simulink model "Rover"  (R2023b)
settings: Solver=FixedStepDiscrete  StartTime=0.0  StopTime=1000  RelTol=1e-3  EnableMultiTasking=on
model workspace (MAT data in the model file):
  state_1 = 0
(part 2 of 2)

== stateflow chart Rover/Chart ==
  settings: updateMethod=DISCRETE  sampleTime=0.001
  state BOARD_1 [parallel]
    settings: executionOrder=1
    state WAITING_INITIALIZATION
      en:
      init_encoder();
      init_encoder();
      init_encoder();
      init_encoder();
      init_motor_driver();
      init_motor_driver();
    state INITIALIZED
    state WORKING
      state LED_CONTROLLER [parallel]
        settings: executionOrder=3
        state SINGLE
          state RIGHT [parallel]
            settings: executionOrder=1
            state OFF
            state ON
            (default) -> BOARD_1.WORKING.LED_CONTROLLER.SINGLE.RIGHT.OFF
            BOARD_1.WORKING.LED_CONTROLLER.SINGLE.RIGHT.ON -> BOARD_1.WORKING.LED_CONTROLLER.SINGLE.RIGHT.OFF : [RH_LED_OFF]
                | {rh_led.off()}
            BOARD_1.WORKING.LED_CONTROLLER.SINGLE.RIGHT.OFF -> BOARD_1.WORKING.LED_CONTROLLER.SINGLE.RIGHT.ON : [RH_LED_ON]
                | {rh_led.on()}
          state LEFT [parallel]
            settings: executionOrder=2
            state OFF
            state ON
            (default) -> BOARD_1.WORKING.LED_CONTROLLER.SINGLE.LEFT.OFF
            BOARD_1.WORKING.LED_CONTROLLER.SINGLE.LEFT.ON -> BOARD_1.WORKING.LED_CONTROLLER.SINGLE.LEFT.OFF : [LH_LED_OFF]
                | {lh_led.off()}
            BOARD_1.WORKING.LED_CONTROLLER.SINGLE.LEFT.OFF -> BOARD_1.WORKING.LED_CONTROLLER.SINGLE.LEFT.ON : [LH_LED_ON]
                | {lh_led.on()}
        state rh_led [group]
        state BOTH
          state WAITING_ON
          state ON
            en:
            rh_led.on();
            lh_led.on()
          state WAITING_OFF
          (default) -> WAITING_ON
          WAITING_ON -> BOARD_1.WORKING.LED_CONTROLLER.BOTH.ON : [LEDS_BTN_RELEASED]
          BOARD_1.WORKING.LED_CONTROLLER.BOTH.ON -> WAITING_OFF : [LEDS_BTN_PRESSED]
        state lh_led [group]
        (default) -> SINGLE
        SINGLE -> BOTH : [LEDS_BTN_PRESSED]
        WAITING_OFF -> SINGLE : [LEDS_BTN_RELEASED]
            | {rh_led.off(); lh_led.off()}
      state STATE_UPDATING [parallel]
        settings: executionOrder=1
        state UPDATE
          en:
          rpm_motors = read_rpm();
          motors_direction = read_motors_direction();
          temperature_B1 = read_temperature();
        (default) -> BOARD_1.WORKING.STATE_UPDATING.UPDATE
        BOARD_1.WORKING.STATE_UPDATING.UPDATE -> BOARD_1.WORKING.STATE_UPDATING.UPDATE : after(READ_PERIOD,  msec)
      state COMM_PROCESS_DECISION [parallel]
        settings: executionOrder=2
        state WAITING_FOR_RTR [parallel]
          settings: executionOrder=2
          state WAITING_BOARD_2
          state BOARD_2_READY
          (default) -> WAITING_BOARD_2
          WAITING_BOARD_2 -> BOARD_2_READY : [B2_RTR]
          BOARD_2_READY -> WAITING_BOARD_2 : [RESET]
        state COMMUNICATION [parallel]
          settings: executionOrder=1
          state TRANSMITTING_TO_B2_1
            en:
            B1_state = capture_state(rpm_motors, motors_direction, ...
            temperature_B1);
          state WAITING_B2_RTR_1
            en: has_retransmitted = false;
          state WAITING_B2_TRANSMISSION_1
            en: send(B1_RTR, BOARD_2)
          state PROCESSING
            en:
            encoder_status = check_encoder(rpm_motors);
            motor_driver_status = check_temperature(check_temperature_values(temperature_B1, temperature_B2));
            mpu_status = check_mpu(control_value, MPU_MASK);
            joypad_status = check_joypad(control_value, JOYPAD_MASK);
            sabertooth_status = check_motor_driver(motors_direction, current_state);
          state res = check_temperature(temperature_status) [function]
            (default) -> (junction 3062)
            (junction 3062) -> (junction 3053) [order 1] : [temperature_status == TEMPERATURE_STATUS.CRITICAL]
                | {res = TEMPERATURE_STATUS.CRITICAL;
                | temperature_out = 2;}
            (junction 3062) -> (junction 3063) [order 2] : [temperature_status == TEMPERATURE_STATUS.NORMAL && ...
                | (in(TEMPERATURE_CONTROLLER.TIMER_STARTED) || ...
                | in(TEMPERATURE_CONTROLLER.TIMER_ELAPSED))]
                | {send(RESET_TEMP_TIMER, TEMPERATURE_CONTROLLER);
                | res = TEMPERATURE_STATUS.NORMAL;
                | temperature_out = 0;}
            (junction 3062) -> (junction 3051) [order 3]
            (junction 3051) -> (junction 3067) [order 1] : [in(TEMPERATURE_CONTROLLER.TIMER_ELAPSED)]
                | {res =TEMPERATURE_STATUS.ABOVE_NORMAL;
                | temperature_out = 1;}
            (junction 3051) -> (junction 3055) [order 2] : [temperature_status == TEMPERATURE_STATUS.ABOVE_NORMAL && ...
                | in(TEMPERATURE_CONTROLLER.TIMER_STOP)]
                | {send(START_TEMP_TIMER, TEMPERATURE_CONTROLLER);
                | res = TEMPERATURE_STATUS.NORMAL;
                | temperature_out = 0;}
            (junction 3051) -> (junction 3056) [order 3] : {res = TEMPERATURE_STATUS.NORMAL;
                | temperature_out = 0;}
          state WAITING_B2_RTR_2
          state TRANSMITTING_TO_B2_2
            en: B1_intention = [double(next_state), ...
            double(degraded), double(braking)];
          state WAITING_B2_TRANSMISSION_2
            en: send(B1_RTR, BOARD_2)
          (junction 1462) -> TRANSMITTING_TO_B2_1 [order 2] : [~has_retransmitted]/{has_retransmitted = true;}
          (default) -> WAITING_B2_RTR_1
          WAITING_B2_RTR_1 -> TRANSMITTING_TO_B2_1 [order 1] : [in(WAITING_FOR_RTR.BOARD_2_READY)]
              | {send(RESET, WAITING_FOR_RTR)}
          TRANSMITTING_TO_B2_1 -> (junction 1462) [order 2] : after(COMM_TIMEOUT,msec)
          (junction 1462) -> (junction 3045) [order 1] : [has_retransmitted]
          (junction 1483) -> (junction 1462) [order 2]
          (junction 3045) -> (junction 1482)
          WAITING_B2_RTR_1 -> (junction 1484) [order 2] : after(B2_ALIVE, msec)
          (junction 3049) -> WAITING_B2_RTR_1
          TRANSMITTING_TO_B2_1 -> WAITING_B2_TRANSMISSION_1 [order 1] : [B2_ACK]{has_retransmitted = false;}
          WAITING_B2_TRANSMISSION_1 -> (junction 1482) [order 1] : after(COMM_TIMEOUT, msec)
          (junction 1482) -> (junction 3047)
          WAITING_B2_TRANSMISSION_1 -> BOARD_1.WORKING.COMM_PROCESS_DECISION.COMMUNICATION.PROCESSING [order 2] : [change(B2_state)]
              | {[obstacle_distances, accX, gyroZ, y_analog, x_analog, control_buttons, ...
              |     control_value, temperature_B2] = update_global_state(B2_state);
              | send(B1_ACK, BOARD_2)}
          BOARD_1.WORKING.COMM_PROCESS_DECISION.COMMUNICATION.PROCESSING -> (junction 1879)
          (junction 1879) -> (junction 1878) [order 1] : [encoder_status == ENCODER_STATUS.ENCODER_ERR || ...
              | joypad_status == JOYPAD_ERR || ...
              | sabertooth_status == SABERTOOTH_STATUS.SABERTOOTH_ERR || ...
              | motor_driver_status == TEMPERATURE_STATUS.CRITICAL]
              | {next_state = EMERGENCY;}
          (junction 1879) -> (junction 1886) [order 2]
          (junction 1878) -> (junction 1877)
          (junction 1886) -> (junction 1885) [order 1] : [(encoder_status ~= ENCODER_STATUS.ENCODER_ERR  && ...
              | encoder_status ~= ENCODER_STATUS.ENCODER_OK) || ...
              | mpu_status == MPU_STATUS.MPU_ERR || ...
              | motor_driver_status == TEMPERATURE_STATUS.ABOVE_NORMAL]
              | {degraded = DEGRADED_STATUS.ACTIVE;}
          (junction 1886) -> (junction 1882) [order 2]
          (junction 1885) -> (junction 1884)
          (junction 1882) -> (junction 1884) : {degraded = DEGRADED_STATUS.INACTIVE;}
          (junction 1884) -> (junction 1877) : {next_state = update_next_state(current_state, y_analog, ...
              |         x_analog, obstacle_distances, control_buttons);}
          (junction 1877) -> WAITING_B2_RTR_2
          WAITING_B2_RTR_2 -> (junction 3047) [order 1] : after(COMM_TIMEOUT, msec)
          (junction 3047) -> (junction 3041)
          WAITING_B2_RTR_2 -> TRANSMITTING_TO_B2_2 [order 2] : [in(WAITING_FOR_RTR.BOARD_2_READY)]
              | {send(RESET, WAITING_FOR_RTR)}
          (junction 1483) -> TRANSMITTING_TO_B2_2 [order 1] : [~has_retransmitted]/{has_retransmitted = true;}
          TRANSMITTING_TO_B2_2 -> (junction 1483) [order 2] : after(COMM_TIMEOUT, msec)
          TRANSMITTING_TO_B2_2 -> WAITING_B2_TRANSMISSION_2 [order 1] : [B2_ACK]
          WAITING_B2_TRANSMISSION_2 -> (junction 3041) [order 2] : after(COMM_TIMEOUT, msec)
          (junction 3041) -> (junction 3042)
          WAITING_B2_TRANSMISSION_2 -> (junction 1475) [order 1] : change(B2_intention)
              | {send(B1_ACK, BOARD_2)}
          (junction 1475) -> (junction 3049) [order 1] : [all(B1_intention == B2_intention)]
              | {current_state = ROVER_STATE(B1_intention(1));
              | led.action()}
          (junction 1475) -> (junction 3042) [order 2]
          (junction 3042) -> (junction 1471)
          (junction 1484) -> (junction 1471)
        state TEMPERATURE_CONTROLLER [parallel]
          settings: executionOrder=3
          state TIMER_STOP
          state TIMER_STARTED
          state TIMER_ELAPSED
          (default) -> BOARD_1.WORKING.COMM_PROCESS_DECISION.TEMPERATURE_CONTROLLER.TIMER_STOP
          BOARD_1.WORKING.COMM_PROCESS_DECISION.TEMPERATURE_CONTROLLER.TIMER_STOP -> BOARD_1.WORKING.COMM_PROCESS_DECISION.TEMPERATURE_CONTROLLER.TIMER_STARTED : [START_TEMP_TIMER]
          BOARD_1.WORKING.COMM_PROCESS_DECISION.TEMPERATURE_CONTROLLER.TIMER_STARTED -> BOARD_1.WORKING.COMM_PROCESS_DECISION.TEMPERATURE_CONTROLLER.TIMER_STOP [order 2] : [RESET_TEMP_TIMER]
          BOARD_1.WORKING.COMM_PROCESS_DECISION.TEMPERATURE_CONTROLLER.TIMER_ELAPSED -> BOARD_1.WORKING.COMM_PROCESS_DECISION.TEMPERATURE_CONTROLLER.TIMER_STOP : [RESET_TEMP_TIMER]
          BOARD_1.WORKING.COMM_PROCESS_DECISION.TEMPERATURE_CONTROLLER.TIMER_STARTED -> BOARD_1.WORKING.COMM_PROCESS_DECISION.TEMPERATURE_CONTROLLER.TIMER_ELAPSED [order 1] : [after(TEMP_TIMEOUT, sec)]
        state led [group]
          state rh_led_action [function]
            (default) -> (junction 2941)
            (junction 2941) -> (junction 2942) [order 1] : [bitand(control_buttons, RH_LED_MASK) == 0]
            (junction 2941) -> (junction 2943) [order 2] : {send(RH_LED_ON, ...
                | LED_CONTROLLER)}
            (junction 2942) -> (junction 2944) : {send(RH_LED_OFF, ...
                | LED_CONTROLLER);}
            (junction 2944) -> (junction 2943)
            (junction 2943) -> (junction 2945)
          state lh_led_action [function]
            (default) -> (junction 2955)
            (junction 2955) -> (junction 2946) [order 1] : [bitand(control_buttons, LH_LED_MASK) == 0]
            (junction 2955) -> (junction 2948) [order 2] : {send(LH_LED_ON, ...
                | LED_CONTROLLER)}
            (junction 2946) -> (junction 2949) : {send(LH_LED_OFF, ...
                | LED_CONTROLLER);}
            (junction 2949) -> (junction 2948)
            (junction 2948) -> (junction 2956)
          state action [function]
            (default) -> (junction 2958)
            (junction 2958) -> (junction 2960) [order 1] : [bitand(control_buttons, BOTH_LED_MASK) ~= 0]
            (junction 2958) -> (junction 2964) [order 2] : {send(LEDS_BTN_RELEASED, ...
                | LED_CONTROLLER)}
            (junction 2960) -> (junction 2962) : {send(LEDS_BTN_PRESSED, ...
                | LED_CONTROLLER)}
            (junction 2962) -> (junction 2964)
            (junction 2964) -> (junction 2967) : {rh_led_action();
                | lh_led_action()}
    state EMERGENCY
      en:
      rover_status_out = 2;
      % fermare i motori
    (default) -> BOARD_1.WAITING_INITIALIZATION
    BOARD_1.WAITING_INITIALIZATION -> BOARD_1.INITIALIZED : after(1, msec)
    BOARD_1.INITIALIZED -> BOARD_1.WORKING : [in(BOARD_2.INITIALIZED) || in(BOARD_2.WORKING)]
    (junction 1471) -> BOARD_1.EMERGENCY
  state BOARD_2 [parallel]
    settings: executionOrder=2
    state WAITING_INITIALIZATION
      en:
      init_motor_driver();
      init_motor_driver();
      init_ps2x();
      init_ultrasonic_sensors();
      init_mpu();
    state INITIALIZED
    state WORKING
      state STATE_UPDATING [parallel]
        settings: executionOrder=1
        state UPDATE
          en:
          obstacle_distances = read_ultrasonic_sensors();
          [accX, gyroZ] = read_mpu();
          [y_analog, x_analog, control_buttons, control_value] = read_joypad(control_buttons);
          temperature_B2 = read_temperature();
        (default) -> BOARD_2.WORKING.STATE_UPDATING.UPDATE
        BOARD_2.WORKING.STATE_UPDATING.UPDATE -> BOARD_2.WORKING.STATE_UPDATING.UPDATE : after(READ_PERIOD, msec)
      state EXECUTION [parallel]
        settings: executionOrder=3
        state DRIVE
          state MODE [parallel]
            settings: executionOrder=1
            state NORMAL
              en:
              rover_status_out = 0;
              % settare velocità
              % massima
            state DEGRADED
              en:
              rover_status_out = 1;
              % settare velocità
              % massima
            (default) -> NORMAL
            DEGRADED -> NORMAL : [MINOR_ERROR_RES]
            NORMAL -> DEGRADED : [MINOR_ERROR]
          state EXECUTE [parallel]
            settings: executionOrder=2
            state MOVE
              state STOP
                state SMOOTH_STOP
                  en:
                  stop.smooth()
                state HARD_STOP
                  state BRAKE
                    en:
                    stop.hard()
                  state ROTATION
                    state ROTATE_RIGHT
                      en:
                      go.right()
                    state ROTATE_LEFT
                      en:
                      go.left()
                    (default) -> (junction 2721)
                    (junction 2721) -> ROTATE_RIGHT [order 1] : [obstacle ~= OBSTACLE_DIR.RIGHT_SIDE]
                    (junction 2721) -> ROTATE_LEFT [order 2]
                  (junction 2736) -> BRAKE [order 2]
                  (default) -> (junction 2736)
                  (junction 2736) -> BOARD_2.WORKING.EXECUTION.DRIVE.EXECUTE.MOVE.STOP.HARD_STOP.ROTATION [order 1] : [obstacle ~= OBSTACLE_DIR.LEFT_RIGHT && ...
                      | obstacle ~= OBSTACLE_DIR.NOTONE]
                  BOARD_2.WORKING.EXECUTION.DRIVE.EXECUTE.MOVE.STOP.HARD_STOP.ROTATION -> BRAKE : [gyroZ >= 90]
                (default) -> (junction 2730)
                (junction 2730) -> SMOOTH_STOP [order 1] : [braking == SMOOTH]
                (junction 2730) -> HARD_STOP [order 2]
              state BACKWARD
                en:
                go.backward()
              state FORWARD
                en:
                go.ahead()
              state FORWARD_RIGHT
                en:
                go.forward_right()
              state FORWARD_LEFT
                en:
                go.forward_left()
              state RIGHT
                en:
                go.right()
              state LEFT
                en:
                go.left()
              state ALT_BACKWARD
                state ROTATION
                  en:
                  go.right();
                state ROTATED
                  en:
                  stop.hard();
                  control_buttons = 0
                BOARD_2.WORKING.EXECUTION.DRIVE.EXECUTE.MOVE.ALT_BACKWARD.ROTATION -> ROTATED : [gyroZ >= 180]
                (default) -> BOARD_2.WORKING.EXECUTION.DRIVE.EXECUTE.MOVE.ALT_BACKWARD.ROTATION
            state IDLE
            (junction 1424) -> (junction 1425)
            (junction 1425) -> IDLE
            STOP -> (junction 1424) : [all(rpm_motors == 0)]
            (default) -> IDLE
            MOVE -> (junction 1420)
            (junction 1420) -> (junction 1415)
            IDLE -> (junction 1413)
            (junction 1415) -> STOP [order 1] : [IDLE]
            (junction 1415) -> (junction 1427) [order 2]
            (junction 1413) -> (junction 1427)
            (junction 1427) -> BACKWARD [order 1] : [BACKWARD]
            (junction 1427) -> (junction 1414) [order 2]
            (junction 1414) -> FORWARD [order 1] : [FORWARD]
            (junction 1414) -> (junction 1421) [order 2]
            (junction 1421) -> (junction 2085) [order 1] : [FORWARD_RIGHT]
            (junction 2085) -> FORWARD_RIGHT [order 2]
            (junction 1421) -> (junction 1432) [order 2]
            (junction 2085) -> (junction 2087) [order 1] : [in(MODE.DEGRADED)]
            (junction 1432) -> (junction 2090) [order 1] : [FORWARD_LEFT]
            (junction 2090) -> FORWARD_LEFT [order 2]
            (junction 1432) -> (junction 1428) [order 2]
            (junction 2090) -> (junction 2092) [order 1] : [in(MODE.DEGRADED)]
            (junction 1428) -> (junction 2087) [order 1] : [RIGHT]
            (junction 2087) -> BOARD_2.WORKING.EXECUTION.DRIVE.EXECUTE.MOVE.RIGHT
            (junction 1428) -> (junction 1408) [order 2]
            (junction 1408) -> (junction 2092) [order 1] : [LEFT]
            (junction 2092) -> BOARD_2.WORKING.EXECUTION.DRIVE.EXECUTE.MOVE.LEFT
            (junction 1408) -> (junction 2675) [order 2]
            (junction 2675) -> ALT_BACKWARD : [ALT_BACKWARD]
          state go [group]
          state stop [group]
      state COMM_PROCESS_DECISION [parallel]
        settings: executionOrder=2
        state COMMUNICATION [parallel]
          settings: executionOrder=1
          state WAITING_FOR_COMMUNICATION
            en: has_retransmitted = false;
          state WAITING_B1_TRANSMISSION_1
            en: send(B2_RTR, BOARD_1)
          state WAITING_B1_RTR_1
            en:
            [rpm_motors, motors_direction, temperature_B1] = update_global_state(B1_state);
          state res = check_temperature(temperature_status) [function]
            (default) -> (junction 2144)
            (junction 2144) -> (junction 2143) [order 1] : [temperature_status == TEMPERATURE_STATUS.CRITICAL]
                | {res = TEMPERATURE_STATUS.CRITICAL;
                | temperature_out = 2;}
            (junction 2144) -> (junction 2546) [order 2] : [temperature_status == TEMPERATURE_STATUS.NORMAL && ...
                | (in(TEMPERATURE_CONTROLLER.TIMER_STARTED) || ...
                | in(TEMPERATURE_CONTROLLER.TIMER_ELAPSED))]
                | {send(RESET_TEMP_TIMER, TEMPERATURE_CONTROLLER);
                | res = TEMPERATURE_STATUS.NORMAL;
                | temperature_out = 0;}
            (junction 2144) -> (junction 2138) [order 3]
            (junction 2138) -> (junction 2134) [order 1] : [in(TEMPERATURE_CONTROLLER.TIMER_ELAPSED)]
                | {res =TEMPERATURE_STATUS.ABOVE_NORMAL;
                | temperature_out = 1;}
            (junction 2138) -> (junction 2145) [order 2] : [temperature_status == TEMPERATURE_STATUS.ABOVE_NORMAL && ...
                | in(TEMPERATURE_CONTROLLER.TIMER_STOP)]
                | {send(START_TEMP_TIMER, TEMPERATURE_CONTROLLER);
                | res = TEMPERATURE_STATUS.NORMAL;
                | temperature_out = 0;}
            (junction 2138) -> (junction 2139) [order 3] : {res = TEMPERATURE_STATUS.NORMAL;
                | temperature_out = 0;}
          state TRANSMITTING_TO_B1_1
            en:
            B2_state  = capture_state(obstacle_distances, accX, gyroZ, y_analog, ...
            x_analog, control_buttons, control_value, temperature_B2);
          state PROCESSING
            en:
            encoder_status = check_encoder(rpm_motors);
            temperature_status = check_temperature(check_temperature_values(temperature_B1, temperature_B2));
            mpu_status = check_mpu(control_value, MPU_MASK);
            joypad_status = check_joypad(control_value, JOYPAD_MASK);
            motor_driver_status = check_motor_driver(motors_direction, current_state);
          state WAITING_B1_TRANSMISSION_2
            en: send(B2_RTR, BOARD_1)
          state WAITING_B1_RTR_2
            en:
            if degraded == DEGRADED_STATUS.ACTIVE
            send(MINOR_ERROR, EXECUTION)
            else
            send(MINOR_ERROR_RES, EXECUTION)
            end
            current_state = next_state;
            action
          state COMMUNICATION_TIMEOUT
          state TRANSMITTING_TO_B1_2
            en: B2_intention = [double(next_state), ...
            double(degraded), double(braking)];
          (default) -> WAITING_FOR_COMMUNICATION
          WAITING_B1_TRANSMISSION_1 -> (junction 1528) [order 2] : after(COMM_TIMEOUT, msec)
          WAITING_FOR_COMMUNICATION -> WAITING_B1_TRANSMISSION_1 : [after(COMM_PERIOD, msec)]
          (junction 1528) -> (junction 3070)
          WAITING_B1_TRANSMISSION_1 -> WAITING_B1_RTR_1 [order 1] : [change(B1_state)]
              | {send(B2_ACK, BOARD_1)}
          (junction 3078) -> WAITING_FOR_COMMUNICATION
          WAITING_B1_RTR_1 -> (junction 3070) [order 1] : after(COMM_TIMEOUT, msec)
          (junction 3070) -> (junction 1529)
          WAITING_B1_RTR_1 -> TRANSMITTING_TO_B1_1 [order 2] : [in(WAITING_FOR_RTR.BOARD_1_READY)]
              | {send(RESET, WAITING_FOR_RTR)}
          (junction 1509) -> TRANSMITTING_TO_B1_1 [order 1] : [~has_retransmitted]{has_retransmitted = true;}
          TRANSMITTING_TO_B1_1 -> (junction 1509) [order 2] : after(COMM_TIMEOUT, msec)
          (junction 1509) -> (junction 3074) [order 2] : [has_retransmitted]
          TRANSMITTING_TO_B1_1 -> BOARD_2.WORKING.COMM_PROCESS_DECISION.COMMUNICATION.PROCESSING [order 1] : [B1_ACK]{has_retransmitted = false;}
          BOARD_2.WORKING.COMM_PROCESS_DECISION.COMMUNICATION.PROCESSING -> (junction 1729)
          (junction 1729) -> (junction 1731) [order 1] : [encoder_status == ENCODER_STATUS.ENCODER_ERR || ...
              | joypad_status == JOYPAD_STATUS.JOYPAD_ERR || ...
              | motor_driver_status == SABERTOOTH_STATUS.SABERTOOTH_ERR || ...
              | temperature_status == TEMPERATURE_STATUS.CRITICAL]
              | {next_state = EMERGENCY;}
          (junction 1729) -> (junction 1733) [order 2]
          (junction 1731) -> (junction 1744)
          (junction 1733) -> (junction 1735) [order 1] : [(encoder_status ~= ENCODER_STATUS.ENCODER_ERR  && ...
              | encoder_status ~= ENCODER_STATUS.ENCODER_OK) || ...
              | mpu_status == MPU_STATUS.MPU_ERR || ...
              | temperature_status == TEMPERATURE_STATUS.ABOVE_NORMAL]
              | {degraded = DEGRADED_STATUS.ACTIVE;}
          (junction 1733) -> (junction 1738) [order 2]
          (junction 1735) -> (junction 1740)
          (junction 1738) -> (junction 1740) : {degraded = DEGRADED_STATUS.INACTIVE;}
          (junction 1740) -> (junction 1744) : {next_state = update_next_state(current_state, y_analog, ...
              |         x_analog, obstacle_distances, control_buttons);
              | obstacle = nearby_obstacle_direction(obstacle_distances);}
          (junction 1744) -> WAITING_B1_TRANSMISSION_2
          WAITING_B1_TRANSMISSION_2 -> (junction 3074) [order 1] : after(COMM_TIMEOUT, msec)
          (junction 3074) -> (junction 1501)
          WAITING_B1_TRANSMISSION_2 -> (junction 2076) [order 2] : [change(B1_intention)]
              | {send(B2_ACK, BOARD_1)}
          (junction 2076) -> (junction 3068) [order 1] : [all(B1_intention ~= [double(next_state), double(degraded), ...
              | double(braking)]) || next_state == EMERGENCY]
          (junction 2076) -> WAITING_B1_RTR_2 [order 2]
          WAITING_B1_RTR_2 -> (junction 1501) [order 1] : [after(COMM_TIMEOUT, msec)]
          (junction 1529) -> (junction 1501)
          (junction 3076) -> (junction 1501)
          (junction 1501) -> COMMUNICATION_TIMEOUT : {send(ACTIVE, SINGLE_BOARD);
              | send(MINOR_ERROR, EXECUTION)}
          (junction 1505) -> (junction 3076) [order 2]
          WAITING_B1_RTR_2 -> TRANSMITTING_TO_B1_2 [order 2] : [in(WAITING_FOR_RTR.BOARD_1_READY)]
              | {send(RESET, WAITING_FOR_RTR)}
          TRANSMITTING_TO_B1_2 -> (junction 1505) [order 2] : after(COMM_TIMEOUT, msec)
          (junction 1505) -> TRANSMITTING_TO_B1_2 [order 1] : [~has_retransmitted]{has_retransmitted = true;}
          TRANSMITTING_TO_B1_2 -> (junction 3078) [order 1] : [B1_ACK]
        state WAITING_FOR_RTR [parallel]
          settings: executionOrder=2
          state WAITING_BOARD_1
          state BOARD_1_READY
          (default) -> WAITING_BOARD_1
          WAITING_BOARD_1 -> BOARD_1_READY : [B1_RTR]
          BOARD_1_READY -> WAITING_BOARD_1 : [RESET]
        state TEMPERATURE_CONTROLLER [parallel]
          settings: executionOrder=3
          state TIMER_STOP
          state TIMER_STARTED
          state TIMER_ELAPSED
          (default) -> BOARD_2.WORKING.COMM_PROCESS_DECISION.TEMPERATURE_CONTROLLER.TIMER_STOP
          BOARD_2.WORKING.COMM_PROCESS_DECISION.TEMPERATURE_CONTROLLER.TIMER_STOP -> BOARD_2.WORKING.COMM_PROCESS_DECISION.TEMPERATURE_CONTROLLER.TIMER_STARTED : [START_TEMP_TIMER]
          BOARD_2.WORKING.COMM_PROCESS_DECISION.TEMPERATURE_CONTROLLER.TIMER_STARTED -> BOARD_2.WORKING.COMM_PROCESS_DECISION.TEMPERATURE_CONTROLLER.TIMER_STOP [order 2] : [RESET_TEMP_TIMER]
          BOARD_2.WORKING.COMM_PROCESS_DECISION.TEMPERATURE_CONTROLLER.TIMER_ELAPSED -> BOARD_2.WORKING.COMM_PROCESS_DECISION.TEMPERATURE_CONTROLLER.TIMER_STOP : [RESET_TEMP_TIMER]
          BOARD_2.WORKING.COMM_PROCESS_DECISION.TEMPERATURE_CONTROLLER.TIMER_STARTED -> BOARD_2.WORKING.COMM_PROCESS_DECISION.TEMPERATURE_CONTROLLER.TIMER_ELAPSED [order 1] : [after(TEMP_TIMEOUT, sec)]
      state action [function]
        (default) -> (junction 2798)
        (junction 2798) -> (junction 2799) [order 1] : [current_state == ROVER_STATE.IDLE]
        (junction 2798) -> (junction 2825) [order 2]
        (junction 2799) -> (junction 2833) : {send(IDLE, EXECUTION);}
        (junction 2833) -> (junction 2813)
        (junction 2813) -> (junction 2803)
        (junction 2825) -> (junction 2816) [order 1] : [current_state == ROVER_STATE.FORWARD]
        (junction 2825) -> (junction 2810) [order 2]
        (junction 2816) -> (junction 2802) : {send(FORWARD, EXECUTION);}
        (junction 2802) -> (junction 2803)
        (junction 2803) -> (junction 2807)
        (junction 2810) -> (junction 2827) [order 1] : [current_state == ROVER_STATE.LEFT]
        (junction 2810) -> (junction 2821) [order 2]
        (junction 2827) -> (junction 2801) : {send(LEFT, EXECUTION);}
        (junction 2801) -> (junction 2807)
        (junction 2807) -> (junction 2819)
        (junction 2821) -> (junction 2818) [order 1] : [current_state == ROVER_STATE.RIGHT]
        (junction 2821) -> (junction 2820) [order 2]
        (junction 2818) -> (junction 2806) : {send(RIGHT, EXECUTION);}
        (junction 2806) -> (junction 2819)
        (junction 2819) -> (junction 2828)
        (junction 2820) -> (junction 2804) [order 1] : [current_state == ROVER_STATE.FORWARD_RIGHT]
        (junction 2820) -> (junction 2826) [order 2]
        (junction 2804) -> (junction 2805) : {send(FORWARD_RIGHT, EXECUTION);}
        (junction 2805) -> (junction 2828)
        (junction 2828) -> (junction 2823)
        (junction 2826) -> (junction 2822) [order 1] : [current_state == ROVER_STATE.FORWARD_LEFT]
        (junction 2826) -> (junction 2811) [order 2]
        (junction 2822) -> (junction 2831) : {send(FORWARD_LEFT, EXECUTION);}
        (junction 2831) -> (junction 2823)
        (junction 2823) -> (junction 2808)
        (junction 2811) -> (junction 2824) [order 1] : [current_state == ROVER_STATE.BACKWARD]
        (junction 2811) -> (junction 2867) [order 2]
        (junction 2824) -> (junction 2817) : {send(BACKWARD, EXECUTION);}
        (junction 2817) -> (junction 2808)
        (junction 2808) -> (junction 2873)
        (junction 2867) -> (junction 2869) [order 1] : [current_state == ROVER_STATE.ALT_BACKWARD]
        (junction 2867) -> (junction 2829) [order 2] : {send(IDLE, EXECUTION);}
        (junction 2869) -> (junction 2871)
        (junction 2871) -> (junction 2873) : {send(ALT_BACKWARD, EXECUTION);}
        (junction 2873) -> (junction 2800)
        (junction 2800) -> (junction 2829)
        (junction 2829) -> (junction 2830)
      state SINGLE_BOARD [parallel]
        settings: executionOrder=4
        state PROCESSING
          en:
          if(temperature_B2 >= CRITICAL_TEMP)
          temperature_status = TEMPERATURE_STATUS.CRITICAL;
          end
          mpu_status =  check_mpu(control_value, MPU_MASK);
          joypad_status = check_joypad(control_value, JOYPAD_MASK);
        state WAITING_START
        state WAITING
          en:
          action
        WAITING_START -> BOARD_2.WORKING.SINGLE_BOARD.PROCESSING : [ACTIVE]% spegnere Board 1
        (default) -> WAITING_START
        WAITING -> BOARD_2.WORKING.SINGLE_BOARD.PROCESSING : [after(COMM_PERIOD, msec)]
        BOARD_2.WORKING.SINGLE_BOARD.PROCESSING -> (junction 2750)
        (junction 2750) -> WAITING [order 2] : {current_state = update_next_state(current_state, y_analog, ...
            |         x_analog, obstacle_distances, control_buttons);
            | obstacle = nearby_obstacle_direction(obstacle_distances);}
      (junction 3068) -> (junction 1843)
      (junction 2750) -> (junction 1843) [order 1] : [mpu_status == MPU_STATUS.MPU_ERR || ...
          | temperature_status == TEMPERATURE_STATUS.CRITICAL || ...
          | joypad_status == JOYPAD_STATUS.JOYPAD_ERR]
      (junction 1843) -> (junction 3085)
      DRIVE -> (junction 3084) : [bitand(control_buttons, EMERGENCY_STOP_MASK) ~= 0]
      (junction 3084) -> (junction 3085)
    state EMERGENCY
      en:
      rover_status_out = 2;
      % spegnere la Board 1
      % fermare i motori
    (default) -> BOARD_2.WAITING_INITIALIZATION
    BOARD_2.WAITING_INITIALIZATION -> BOARD_2.INITIALIZED : after(2, msec)
    BOARD_2.INITIALIZED -> BOARD_2.WORKING : [in(BOARD_1.INITIALIZED) || in(BOARD_1.WORKING)]
    (junction 3085) -> BOARD_2.EMERGENCY
  data: rpm_motors function_output; motors_direction function_output; temperature_B1 function_output; control_value function_input; mpu_status function_output; mask function_input; next_state function_output; current_state function_input; y_analog function_input; x_analog function_input; obstacle_distances function_input; braking function_output; control_buttons function_input; rpm_motors function_input; encoder_status function_output; control_variable function_input; joypad_status function_output; mask function_input; state function_output; rpm_motors function_input; motors_direction function_input; temperature_B1 function_input; temperature_B1 function_input; temperature_status function_output; temperature_B2 function_input; sabertooth_status function_output; motors_direction function_input; current_state function_input; B2_state function_input; obstacle_distances function_output; accX function_output; gyroZ function_output; y_analog function_output; x_analog function_output; control_buttons function_output; control_value function_output; temperature_B2 function_output; temperature_status function_input; res function_output; current_state local Enum: ROVER_STATE =ROVER_STATE.IDLE; next_state local Enum: ROVER_STATE =ROVER_STATE.IDLE; has_retransmitted local boolean =false; braking local Enum: BRAKING_TYPE =BRAKING_TYPE.NONE; rpm_motors local double =[0 0 0 0]; motors_direction local int8 =[0 0]; obstacle_distances local double =[0 0 0]; temperature_B1 local double =0; temperature_B2 local double =0; accX local double =0; gyroZ local double =0; y_analog local int8 =0; x_analog local int8 =0; control_buttons local uint8 =0; control_value local uint8 =0; encoder_status local Enum: ENCODER_STATUS =ENCODER_STATUS.ENCODER_OK; motor_driver_status local Enum: TEMPERATURE_STATUS =TEMPERATURE_STATUS.NORMAL; mpu_status local Enum: MPU_STATUS =MPU_STATUS.MPU_OK; joypad_status local Enum: JOYPAD_STATUS =JOYPAD_STATUS.JOYPAD_OK; sabertooth_status local Enum: SABERTOOTH_STATUS =SABERTOOTH_STATUS.SABERTOOTH_OK; degraded local Enum: DEGRADED_STATUS =DEGRADED_STATUS.INACTIVE; RH_LED_MASK constant uint8 =1; LH_LED_MASK constant uint8 =2; BOTH_LED_MASK constant uint8 =4; obstacle_distances function_output; temperature_B2 function_output; y_analog function_output; x_analog function_output; control_buttons_out function_output; control_value function_output; control_buttons function_input; accX function_output; gyroZ function_output; B1_state function_input; rpm_motors function_output; motors_direction function_output; temperature_B1 function_output; temperature_B1 function_input; temperature_status function_output; temperature_B2 function_input; rpm_motors function_input; encoder_status function_output; state function_output; obstacle_distances function_input; accX function_input; gyroZ function_input; y_analog function_input; x_analog function_input; control_buttons function_input; control_value function_input; temperature_B2 function_input; sabertooth_status function_output; motors_direction function_input; current_state function_input; temperature_status function_input; res function_output; next_state function_output; current_state function_input; y_analog function_input; x_analog function_input; obstacle_distances function_input; braking function_output; control_buttons function_input; obstacle_distances function_input; obstacle function_output; control_value function_input; joypad_status function_output; mask function_input; control_value function_input; mpu_status function_output; mask function_input; has_retransmitted local boolean =false; current_state local Enum: ROVER_STATE =ROVER_STATE.IDLE; braking local Enum: BRAKING_TYPE =BRAKING_TYPE.NONE; rpm_motors local double =[0 0 0 0]; motors_direction local int8 =[0 0]; obstacle_distances local double =[0 0 0]; temperature_B1 local double =0; temperature_B2 local double =0; accX local double =0; gyroZ local double =0; y_analog local int8 =0; x_analog local int8 =0; control_buttons local uint8 =0; control_value local uint8 =0; next_state local Enum: ROVER_STATE =ROVER_STATE.IDLE; encoder_status local Enum: ENCODER_STATUS =ENCODER_STATUS.ENCODER_OK; temperature_status local Enum: TEMPERATURE_STATUS =TEMPERATURE_STATUS.NORMAL; mpu_status local Enum: MPU_STATUS =MPU_STATUS.MPU_OK; joypad_status local Enum: JOYPAD_STATUS =JOYPAD_STATUS.JOYPAD_OK; motor_driver_status local Enum: SABERTOOTH_STATUS =SABERTOOTH_STATUS.SABERTOOTH_OK; degraded local Enum: DEGRADED_STATUS =DEGRADED_STATUS.INACTIVE; EMERGENCY_STOP_MASK local uint8 =32; obstacle local Enum: OBSTACLE_DIR =OBSTACLE_DIR.NOTONE; B1_state local double; COMM_PERIOD constant double =12; DISTANT_OBSTACLE_DISTANCE constant double =3; NEARBY_OBSTACLE_DISTANCE constant double =0.70; B1_intention local =[0 0 0]; COMM_TIMEOUT constant double =3; MIN_NORMAL_TEMP local =0; MAX_NORMAL_TEMP local =35; CRITICAL_TEMP constant double =50; TEMP_TIMEOUT constant double =15; JOYPAD_MASK constant double =2; MPU_MASK constant double =1; B2_state local double; B2_intention local =[0 0 0]; MIN_SIDE_DISTANCE constant double =0.1; B2_ALIVE constant double =15; READ_PERIOD constant double =10; ALT_BACKWARD_MASK constant double =24; motor_dir_right_in input int8; motor_dir_left_in input int8; temperature_B1_in input double; temperature_B2_in input double; obstacle_left_in input double; obstacle_front_in input double; obstacle_right_in input double; y_analog_in input int8; x_analog_in input int8; fl_wheel output uint8 =0; fr_wheel output uint8 =0; rl_wheel output uint8 =0; rr_wheel output uint8 =0; rh_led_out output boolean =0; lh_led_out output boolean =0; rh_led_in input uint8; lh_led_in input uint8; both_led_in input uint8 =0; temperature_out output uint8 =0; rover_status_out output uint8; combo_in input uint8; alt_backward_in input uint8; emergency_stop_in input uint8; gyroZ_in input double; motor_dir_right_out output int8 =DIRECTION.DEFAULT_DIRECTION; motor_dir_left_out output int8 =DIRECTION.DEFAULT_DIRECTION; rpm input double
  events: RH_LED_ON local FUNCTION_CALL_EVENT; RH_LED_OFF local FUNCTION_CALL_EVENT; LH_LED_ON local FUNCTION_CALL_EVENT; LH_LED_OFF local FUNCTION_CALL_EVENT; LEDS_BTN_PRESSED local FUNCTION_CALL_EVENT; LEDS_BTN_RELEASED local FUNCTION_CALL_EVENT; ACTIVE local FUNCTION_CALL_EVENT; IDLE local FUNCTION_CALL_EVENT; FORWARD local FUNCTION_CALL_EVENT; FORWARD_RIGHT local FUNCTION_CALL_EVENT; FORWARD_LEFT local FUNCTION_CALL_EVENT; RIGHT local FUNCTION_CALL_EVENT; LEFT local FUNCTION_CALL_EVENT; BACKWARD local FUNCTION_CALL_EVENT; ALT_BACKWARD local FUNCTION_CALL_EVENT; RESET local FUNCTION_CALL_EVENT; B1_ACK local FUNCTION_CALL_EVENT; B1_RTR local FUNCTION_CALL_EVENT; B2_ACK local FUNCTION_CALL_EVENT; B2_RTR local FUNCTION_CALL_EVENT; MINOR_ERROR local FUNCTION_CALL_EVENT; MINOR_ERROR_RES local FUNCTION_CALL_EVENT; START_TEMP_TIMER local FUNCTION_CALL_EVENT; RESET_TEMP_TIMER local FUNCTION_CALL_EVENT
  function init_encoder:
    | function init_encoder()
    | 
    | end
  function init_motor_driver:
    | function init_motor_driver()
    | 
    | end
  function on:
    | function on
    | 
    | global rh_led_out
    | 
    | rh_led_out = true;
    | 
    | end
  function off:
    | function off
    | 
    | global rh_led_out
    | 
    | rh_led_out = false;
    | 
    | end
  function on:
    | function on
    | 
    | global lh_led_out
    | 
    | lh_led_out = true;
    | 
    | end
  function off:
    | function off
    | 
    | global lh_led_out
    | 
    | lh_led_out = false;
    | 
    | end
  function rpm_motors = read_rpm:
    | function rpm_motors = read_rpm
    | 
    | global rpm
    | 
    | rpm_motors = [rpm, rpm, rpm, rpm];
    | 
    | end
  function motors_direction = read_motors_direction:
    | function motors_direction = read_motors_direction()
    | 
    | global motor_dir_right_in motor_dir_left_in
    | 
    | motors_direction = [motor_dir_left_in, motor_dir_right_in];
    | 
    | end
  function temperature_B1 = read_temperature:
    | function temperature_B1 = read_temperature()
    | 
    | global temperature_B1_in
    | 
    | temperature_B1 = temperature_B1_in;
    | 
    | end
  function mpu_status = check_mpu(control_value, mask):
    | function mpu_status = check_mpu(control_value, mask)
    | 
    | mpu_status = MPU_STATUS.MPU_OK;
    | if bitand(control_value, mask) == 0
    |     mpu_status = MPU_STATUS.MPU_ERR;
    | 
    | end
  function [next_state, braking] = update_next_state(current_state, ...:
    | function [next_state, braking] = update_next_state(current_state, ...
    |                       y_analog, x_analog, obstacle_distances, control_buttons)
    | 
    | braking = BRAKING_TYPE.NONE;
    | next_state = ROVER_STATE.IDLE;
    | 
    | obstacle_left = obstacle_distances(1);
    | obstacle_front = obstacle_distances(2);
    | obstacle_right = obstacle_distances(3);
    | 
    | if y_analog == 0 
    |             
    |     if x_analog > 0 && obstacle_right >= MIN_SIDE_DISTANCE
    |         
    |         next_state = ROVER_STATE.RIGHT;
    | 
    |     elseif x_analog < 0 && obstacle_left >= MIN_SIDE_DISTANCE
    |     
    |         next_state = ROVER_STATE.LEFT;
    | 
    |     else
    |         if bitand(control_buttons, ALT_BACKWARD_MASK) == ALT_BACKWARD_MASK
    |             next_state = ROVER_STATE.ALT_BACKWARD; 
    |         elseif current_state ~= ROVER_STATE.IDLE 
    |             braking = BRAKING_TYPE.HARD;
    |             next_state = ROVER_STATE.IDLE;
    |         else
    |             next_state = ROVER_STATE.IDLE;
    |         end
    | 
    |     end
    | 
    | elseif y_analog < 0
    | 
    |     next_state = ROVER_STATE.BACKWARD;
    | 
    | elseif obstacle_front <= DISTANT_OBSTACLE_DISTANCE 
    |     
    |     if current_state ~= ROVER_STATE.IDLE 
    |         if (obstacle_front <= NEARBY_OBSTACLE_DISTANCE); braking = BRAKING_TYPE.HARD; else; braking = BRAKING_TYPE.SMOOTH;end
    |     end
    |     next_state = ROVER_STATE.IDLE;
    | 
    | elseif x_analog > 0
    |     
    |     if obstacle_right > DISTANT_OBSTACLE_DISTANCE
    | 
    |         next_state = ROVER_STATE.FORWARD_RIGHT;
    | 
    |     else
    |         
    |         braking = BRAKING_TYPE.HARD;
    |         next_state = ROVER_STATE.IDLE;
    | 
    |     end
    | 
    | elseif x_analog < 0
    | 
    |     if obstacle_left > DISTANT_OBSTACLE_DISTANCE
    | 
    |         next_state = ROVER_STATE.FORWARD_LEFT;
    | 
    |     else
    |         
    |         braking = BRAKING_TYPE.HARD;
    |         next_state = ROVER_STATE.IDLE;
    | 
    |     end
    | 
    | elseif y_analog > 0
    | 
    |         next_state = ROVER_STATE.FORWARD;
    | 
    | else 
    |     
    |     braking = BRAKING_TYPE.HARD;
    |     next_state = ROVER_STATE.IDLE;
    | 
    | end
    | 
    | end
  function encoder_status = check_encoder(rpm_motors):
    | function encoder_status = check_encoder(rpm_motors)
    | 
    |     % Verifica che ciascun elemento di rpm_motors non si discosti da almeno 2 di tutti gli altri di un certo valore 'value'.
    |     % Restituisce -1 se più di un elemento si discosta, l'indice dell'elemento che si discosta se è uno solo,
    |     % altrimenti -2 se nessuno si discosta.
    | 
    |     value = 10;
    | 
    |     encoder_status = ENCODER_STATUS.ENCODER_OK; % Nessuno si discosta inizialmente
    |     contatore_discostamenti = 0; % Contatore per il numero di elementi che si discostano
    | 
    |     for i = 1:length(rpm_motors)
    |         elemento = rpm_motors(i);
    |         discostamenti = 0; % Contatore per il numero di elementi che si discostano dall'elemento corrente
    | 
    |         % Conta quanti altri elementi si discostano di 'value'
    |         for j = 1:length(rpm_motors)
    |             if i ~= j && abs(elemento - rpm_motors(j)) >= value
    |                 discostamenti = discostamenti + 1;
    |             end
    |         end
    | 
    |         % Verifica se l'elemento corrente si discosta da almeno 2 altri elementi
    |         if discostamenti >= 2
    |             if contatore_discostamenti == 0
    |                 switch i
    |                     case 1
    |                         encoder_status = ENCODER_STATUS.ENCODER1_ERR;
    |                     case 2
    |                         encoder_status = ENCODER_STATUS.ENCODER2_ERR;
    |                     case 3
    |                         encoder_status = ENCODER_STATUS.ENCODER3_ERR;
    |                     case 4
    |                         encoder_status = ENCODER_STATUS.ENCODER4_ERR;
    |                     otherwise
    |                         encoder_status = ENCODER_STATUS.ENCODER_ERR;
    |                 end
    |                  % Salva l'indice del primo elemento che si discosta
    |             end
    |             contatore_discostamenti = contatore_discostamenti + 1;
    |         end
    |     end
    | 
    |     % Restituisce -1 se più di un elemento si discosta
    |     if contatore_discostamenti > 1
    |         encoder_status = ENCODER_STATUS.ENCODER_ERR;
    |     end
    | 
    | end
  function joypad_status = check_joypad(control_variable, mask):
    | function joypad_status = check_joypad(control_variable, mask)
    | 
    | joypad_status = JOYPAD_STATUS.JOYPAD_OK;
    | if bitand(control_variable, mask) == 0
    |     joypad_status = JOYPAD_STATUS.JOYPAD_ERR;
    | 
    | end
  function state = capture_state(rpm_motors, motors_direction, ...:
    | function state = capture_state(rpm_motors, motors_direction, ...
    |      temperature_B1)
    | 
    | state = [rpm_motors, double(motors_direction), temperature_B1];
    |       
    | end
  function temperature_status = check_temperature_values(temperature_B1, ...:
    | function temperature_status = check_temperature_values(temperature_B1, temperature_B2)
    | 
    | temperature_status = TEMPERATURE_STATUS.NORMAL;
    | 
    | % potrebbe essere utile per capire se uno dei sensori di temperatura
    | % è rotto
    | if(abs(temperature_B1 - temperature_B2) >= 10) 
    | 
    |     temperature_status = TEMPERATURE_STATUS.CRITICAL;
    | 
    | else
    | 
    |     max_temp = max(temperature_B1, temperature_B2);
    |     
    |     if max_temp >= MIN_NORMAL_TEMP && max_temp <= MAX_NORMAL_TEMP
    |     
    |         temperature_status = TEMPERATURE_STATUS.NORMAL;
    |     
    |     elseif max_temp > MAX_NORMAL_TEMP && max_temp < CRITICAL_TEMP
    |     
    |         temperature_status = TEMPERATURE_STATUS.ABOVE_NORMAL;
    |     
    |     elseif max_temp >= CRITICAL_TEMP
    |     
    |         temperature_status = TEMPERATURE_STATUS.CRITICAL;
    |     
    |     end
    | 
    | end
    | 
    | end
  function sabertooth_status = check_motor_driver(motors_direction, current_state):
    | function sabertooth_status = check_motor_driver(motors_direction, current_state)
    | 
    | % sabertooth_status = SABERTOOTH_STATUS.SABERTOOTH_ERR;
    | % 
    | % direction_mot_1 = motors_direction(1);
    | % direction_mot_2 = motors_direction(2);
    | % 
    | % switch current_state
    | %     case ROVER_STATE.FORWARD
    | %         if direction_mot_1 == DIRECTION.FORWARD_DIRECTION && direction_mot_2 == DIRECTION.FORWARD_DIRECTION
    | %             sabertooth_status = SABERTOOTH_STATUS.SABERTOOTH_OK;
    | %         end
    | %     case ROVER_STATE.BACKWARD
    | %         if direction_mot_1 == DIRECTION.BACKWARD_DIRECTION && direction_mot_2 == DIRECTION.BACKWARD_DIRECTION
    | %             sabertooth_status = SABERTOOTH_STATUS.SABERTOOTH_OK;
    | %         end
    | %     case {ROVER_STATE.FORWARD_RIGHT, ROVER_STATE.RIGHT, ROVER_STATE.ALT_BACKWARD}
    | %         if direction_mot_1 == DIRECTION.FORWARD_DIRECTION && direction_mot_2 == DIRECTION.BACKWARD_DIRECTION
    | %             sabertooth_status = SABERTOOTH_STATUS.SABERTOOTH_OK;
    | %         end
    | %     case {ROVER_STATE.FORWARD_LEFT, ROVER_STATE.LEFT}
    | %         if direction_mot_1 == DIRECTION.BACKWARD_DIRECTION && direction_mot_2 == DIRECTION.FORWARD_DIRECTION
    | %             sabertooth_status = SABERTOOTH_STATUS.SABERTOOTH_OK;
    | %         end
    | %     case ROVER_STATE.IDLE
    | %         if all(rpm_motors == 0)
    | %             if direction_mot_1 == DIRECTION.DEFAULT_DIRECTION && direction_mot_2 == DIRECTION.DEFAULT_DIRECTION
    | %                 sabertooth_status = SABERTOOTH_STATUS.SABERTOOTH_OK;
    | %             end
    | %         elseif obstacle == OBSTACLE_DIR.LEFT_SIDE || obstacle == OBSTACLE_DIR.FRONT
    | %             if direction_mot_1 == DIRECTION.FORWARD_DIRECTION && direction_mot_2 == DIRECTION.BACKWARD_DIRECTION
    | %                     sabertooth_status = SABERTOOTH_STATUS.SABERTOOTH_OK;
    | %             end
    | %         elseif obstacle == OBSTACLE_DIR.RIGHT_SIDE 
    | %             if direction_mot_1 == DIRECTION.BACKWARD_DIRECTION && direction_mot_2 == DIRECTION.FORWARD_DIRECTION
    | %                     sabertooth_status = SABERTOOTH_STATUS.SABERTOOTH_OK;
    | %             end
    | %         else
    | %             sabertooth_status = SABERTOOTH_STATUS.SABERTOOTH_OK;
    | %         end
    | % 
    | %     otherwise
    | %         sabertooth_status = SABERTOOTH_STATUS.SABERTOOTH_ERR;
    | % end
    | 
    | sabertooth_status = SABERTOOTH_STATUS.SABERTOOTH_OK;
    | 
    | end
  function [obstacle_distances, accX, gyroZ, y_analog, x_analog, control_buttons, ...:
    | function [obstacle_distances, accX, gyroZ, y_analog, x_analog, ...
    |     control_buttons, control_value, temperature_B2] = update_global_state(B2_state)
    | 
    | obstacle_distances = [B2_state(1), B2_state(2), B2_state(3)];
    | accX = B2_state(4); gyroZ = B2_state(5);
    | y_analog = int8(B2_state(6)); x_analog = int8(B2_state(7));
    | control_buttons = uint8(B2_state(8)); control_value = uint8(B2_state(9));
    | temperature_B2 = B2_state(10);
    | 
    | end
  function init_mpu:
    | function init_mpu
    | 
    | end
  function init_ps2x:
    | function init_ps2x
    | 
    | end
  function init_ultrasonic_sensors:
    | function init_ultrasonic_sensors
    | 
    | end
  function init_motor_driver:
    | function init_motor_driver
    | 
    | end
  function obstacle_distances = read_ultrasonic_sensors:
    | function obstacle_distances = read_ultrasonic_sensors()
    | 
    | global obstacle_left_in obstacle_front_in obstacle_right_in
    | 
    | obstacle_distances = [obstacle_left_in, obstacle_front_in, obstacle_right_in];
    | 
    | end
  function temperature_B2 = read_temperature:
    | function temperature_B2 = read_temperature()
    | 
    | global temperature_B2_in
    | 
    | temperature_B2 = temperature_B2_in;
    | 
    | end
  function [y_analog, x_analog, control_buttons_out, control_value] = read_joypad(control_buttons):
    | function [y_analog, x_analog, control_buttons_out, control_value] = read_joypad(control_buttons)
    | 
    | global x_analog_in y_analog_in 
    | global rh_led_in lh_led_in both_led_in
    | global combo_in alt_backward_in emergency_stop_in
    | 
    | y_analog = y_analog_in;
    | x_analog = x_analog_in;
    | 
    | lh_led_in_tmp = bitshift(lh_led_in, 1);
    | both_led_in_tmp = bitshift(both_led_in, 2);
    | combo_in_tmp = bitshift(combo_in, 3);
    | alt_backward_in_tmp = bitshift(alt_backward_in, 4);
    | emergency_stop_in_tmp = bitshift(emergency_stop_in, 5);
    | 
    | tmp_and = bitor(lh_led_in_tmp, bitor(both_led_in_tmp, bitor(emergency_stop_in_tmp, bitor(rh_led_in, bitor(bitshift(1, 3), bitshift(1, 4))))));
    | control_buttons_out = bitand(uint8(control_buttons), tmp_and);
    | tmp_or = bitor(lh_led_in_tmp, bitor(both_led_in_tmp, bitor(emergency_stop_in_tmp, bitor(rh_led_in, bitor(combo_in_tmp, alt_backward_in_tmp)))));
    | control_buttons_out = bitor(uint8(control_buttons_out), tmp_or);
    | 
    | control_value = uint8(255);
    | 
    | end
  function [accX, gyroZ] = read_mpu:
    | function [accX, gyroZ] = read_mpu
    | 
    | global gyroZ_in
    | 
    | accX = 0;
    | gyroZ = gyroZ_in;
    | 
    | end
  function ahead:
    | function ahead
    | 
    | global fr_wheel fl_wheel rl_wheel rr_wheel
    | global motor_dir_right_out motor_dir_left_out
    | 
    | fr_wheel = uint8(1);
    | fl_wheel = uint8(1);
    | rl_wheel = uint8(1);
    | rr_wheel = uint8(1);
    | 
    | motor_dir_right_out = int8(2);
    | motor_dir_left_out = int8(2);
    | 
    | end
  function backward:
    | function backward
    | 
    | global fr_wheel fl_wheel rl_wheel rr_wheel
    | global motor_dir_right_out motor_dir_left_out
    | 
    | fr_wheel = uint8(2);
    | fl_wheel = uint8(2);
    | rl_wheel = uint8(2);
    | rr_wheel = uint8(2);
    | 
    | motor_dir_right_out = int8(1);
    | motor_dir_left_out = int8(1);
    | 
    | end
  function forward_right:
    | function forward_right
    | 
    | global fr_wheel fl_wheel rl_wheel rr_wheel
    | global motor_dir_right_out motor_dir_left_out
    | 
    | fr_wheel = uint8(3);
    | fl_wheel = uint8(1);
    | rl_wheel = uint8(1);
    | rr_wheel = uint8(3);
    | 
    | motor_dir_right_out = int8(1);
    | motor_dir_left_out = int8(2);
    | 
    | end
  function forward_left:
    | function forward_left
    | 
    | global fr_wheel fl_wheel rl_wheel rr_wheel
    | global motor_dir_right_out motor_dir_left_out
    | 
    | fr_wheel = uint8(1);
    | fl_wheel = uint8(3);
    | rl_wheel = uint8(3);
    | rr_wheel = uint8(1);
    | 
    | motor_dir_right_out = int8(2); 
    | motor_dir_left_out = int8(1);
    | 
    | end
  function right:
    | function right
    | 
    | global fr_wheel fl_wheel rl_wheel rr_wheel
    | global motor_dir_right_out motor_dir_left_out
    | 
    | fr_wheel = uint8(2);
    | fl_wheel = uint8(1);
    | rl_wheel = uint8(1);
    | rr_wheel = uint8(2);
    | 
    | motor_dir_right_out = int8(1);
    | motor_dir_left_out = int8(2);
    | 
    | end
  function left:
    | function left
    | 
    | global fr_wheel fl_wheel rl_wheel rr_wheel
    | global motor_dir_right_out motor_dir_left_out
    | 
    | fr_wheel = uint8(1);
    | fl_wheel = uint8(2);
    | rl_wheel = uint8(2);
    | rr_wheel = uint8(1);
    | 
    | motor_dir_right_out = int8(2); 
    | motor_dir_left_out = int8(1);
    | 
    | end
  function smooth:
    | function smooth
    | 
    | global fr_wheel fl_wheel rl_wheel rr_wheel
    | global motor_dir_right_out motor_dir_left_out
    | 
    | fr_wheel = uint8(0);
    | fl_wheel = uint8(0);
    | rl_wheel = uint8(0);
    | rr_wheel = uint8(0);
    | 
    | motor_dir_right_out = int8(0);
    | motor_dir_left_out = int8(0);
    | 
    | end
  function hard:
    | function hard
    | 
    | global fr_wheel fl_wheel rl_wheel rr_wheel
    | global motor_dir_right_out motor_dir_left_out
    | 
    | fr_wheel = uint8(0);
    | fl_wheel = uint8(0);
    | rl_wheel = uint8(0);
    | rr_wheel = uint8(0);
    | 
    | motor_dir_right_out = int8(0);
    | motor_dir_left_out = int8(0);
    | 
    | end
  function [rpm_motors, motors_direction, temperature_B1] = update_global_state(B1_state):
    | function [rpm_motors, motors_direction, temperature_B1] = update_global_state(B1_state)
    |  
    | rpm_motors = [B1_state(1), B1_state(2), B1_state(3), B1_state(4)];
    | motors_direction = [int8(B1_state(5)), int8(B1_state(6))];
    | temperature_B1 = B1_state(7);
    | 
    | end
  function temperature_status = check_temperature_values(temperature_B1, ...:
    | function temperature_status = check_temperature_values(temperature_B1, temperature_B2)
    | 
    | temperature_status = TEMPERATURE_STATUS.NORMAL;
    | 
    | % potrebbe essere utile per capire se uno dei sensori di temperatura
    | % è rotto
    | if(abs(temperature_B1 - temperature_B2) >= 10) 
    | 
    |     temperature_status = TEMPERATURE_STATUS.CRITICAL;
    | 
    | else
    | 
    |     max_temp = max(temperature_B1, temperature_B2);
    |     
    |     if max_temp >= MIN_NORMAL_TEMP && max_temp <= MAX_NORMAL_TEMP
    |     
    |         temperature_status = TEMPERATURE_STATUS.NORMAL;
    |     
    |     elseif max_temp > MAX_NORMAL_TEMP && max_temp < CRITICAL_TEMP
    |     
    |         temperature_status = TEMPERATURE_STATUS.ABOVE_NORMAL;
    |     
    |     elseif max_temp >= CRITICAL_TEMP
    |     
    |         temperature_status = TEMPERATURE_STATUS.CRITICAL;
    |     
    |     end
    | 
    | end
    | 
    | end
  function encoder_status = check_encoder(rpm_motors):
    | function encoder_status = check_encoder(rpm_motors)
    | 
    |     % Verifica che ciascun elemento di rpm_motors non si discosti da almeno 2 di tutti gli altri di un certo valore 'value'.
    |     % Restituisce -1 se più di un elemento si discosta, l'indice dell'elemento che si discosta se è uno solo,
    |     % altrimenti -2 se nessuno si discosta.
    | 
    |     value = 10;
    | 
    |     encoder_status = ENCODER_STATUS.ENCODER_OK; % Nessuno si discosta inizialmente
    |     contatore_discostamenti = 0; % Contatore per il numero di elementi che si discostano
    | 
    |     for i = 1:length(rpm_motors)
    |         elemento = rpm_motors(i);
    |         discostamenti = 0; % Contatore per il numero di elementi che si discostano dall'elemento corrente
    | 
    |         % Conta quanti altri elementi si discostano di 'value'
    |         for j = 1:length(rpm_motors)
    |             if i ~= j && abs(elemento - rpm_motors(j)) >= value
    |                 discostamenti = discostamenti + 1;
    |             end
    |         end
    | 
    |         % Verifica se l'elemento corrente si discosta da almeno 2 altri elementi
    |         if discostamenti >= 2
    |             if contatore_discostamenti == 0
    |                 switch i
    |                     case 1
    |                         encoder_status = ENCODER_STATUS.ENCODER1_ERR;
    |                     case 2
    |                         encoder_status = ENCODER_STATUS.ENCODER2_ERR;
    |                     case 3
    |                         encoder_status = ENCODER_STATUS.ENCODER3_ERR;
    |                     case 4
    |                         encoder_status = ENCODER_STATUS.ENCODER4_ERR;
    |                     otherwise
    |                         encoder_status = ENCODER_STATUS.ENCODER_ERR;
    |                 end
    |                  % Salva l'indice del primo elemento che si discosta
    |             end
    |             contatore_discostamenti = contatore_discostamenti + 1;
    |         end
    |     end
    | 
    |     % Restituisce -1 se più di un elemento si discosta
    |     if contatore_discostamenti > 1
    |         encoder_status = ENCODER_STATUS.ENCODER_ERR;
    |     end
    | 
    | end
  function state = capture_state(obstacle_distances, accX, gyroZ, y_analog, ...:
    | function state = capture_state(obstacle_distances, accX, gyroZ, y_analog, ...
    |     x_analog, control_buttons, control_value, temperature_B2)
    | 
    | state = [obstacle_distances, accX, gyroZ, double(y_analog), double(x_analog), ...
    |          double(control_buttons), double(control_value), temperature_B2];
    | 
    | end
  function sabertooth_status = check_motor_driver(motors_direction, current_state):
    | function sabertooth_status = check_motor_driver(motors_direction, current_state)
    | 
    | % sabertooth_status = SABERTOOTH_STATUS.SABERTOOTH_ERR;
    | % 
    | % direction_mot_1 = motors_direction(1);
    | % direction_mot_2 = motors_direction(2);
    | % 
    | % switch current_state
    | %     case ROVER_STATE.FORWARD
    | %         if direction_mot_1 == DIRECTION.FORWARD_DIRECTION && direction_mot_2 == DIRECTION.FORWARD_DIRECTION
    | %             sabertooth_status = SABERTOOTH_STATUS.SABERTOOTH_OK;
    | %         end
    | %     case ROVER_STATE.BACKWARD
    | %         if direction_mot_1 == DIRECTION.BACKWARD_DIRECTION && direction_mot_2 == DIRECTION.BACKWARD_DIRECTION
    | %             sabertooth_status = SABERTOOTH_STATUS.SABERTOOTH_OK;
    | %         end
    | %     case {ROVER_STATE.FORWARD_RIGHT, ROVER_STATE.RIGHT, ROVER_STATE.ALT_BACKWARD}
    | %         if direction_mot_1 == DIRECTION.FORWARD_DIRECTION && direction_mot_2 == DIRECTION.BACKWARD_DIRECTION
    | %             sabertooth_status = SABERTOOTH_STATUS.SABERTOOTH_OK;
    | %         end
    | %     case {ROVER_STATE.FORWARD_LEFT, ROVER_STATE.LEFT}
    | %         if direction_mot_1 == DIRECTION.BACKWARD_DIRECTION && direction_mot_2 == DIRECTION.FORWARD_DIRECTION
    | %             sabertooth_status = SABERTOOTH_STATUS.SABERTOOTH_OK;
    | %         end
    | %     case ROVER_STATE.IDLE
    | %         if all(rpm_motors == 0)
    | %             if direction_mot_1 == DIRECTION.DEFAULT_DIRECTION && direction_mot_2 == DIRECTION.DEFAULT_DIRECTION
    | %                 sabertooth_status = SABERTOOTH_STATUS.SABERTOOTH_OK;
    | %             end
    | %         elseif obstacle == OBSTACLE_DIR.LEFT_SIDE || obstacle == OBSTACLE_DIR.FRONT
    | %             if direction_mot_1 == DIRECTION.FORWARD_DIRECTION && direction_mot_2 == DIRECTION.BACKWARD_DIRECTION
    | %                     sabertooth_status = SABERTOOTH_STATUS.SABERTOOTH_OK;
    | %             end
    | %         elseif obstacle == OBSTACLE_DIR.RIGHT_SIDE 
    | %             if direction_mot_1 == DIRECTION.BACKWARD_DIRECTION && direction_mot_2 == DIRECTION.FORWARD_DIRECTION
    | %                     sabertooth_status = SABERTOOTH_STATUS.SABERTOOTH_OK;
    | %             end
    | %         else
    | %             sabertooth_status = SABERTOOTH_STATUS.SABERTOOTH_OK;
    | %         end
    | % 
    | %     otherwise
    | %         sabertooth_status = SABERTOOTH_STATUS.SABERTOOTH_ERR;
    | % end
    | 
    | sabertooth_status = SABERTOOTH_STATUS.SABERTOOTH_OK;
    | 
    | end
  function [next_state, braking] = update_next_state(current_state, ...:
    | function [next_state, braking] = update_next_state(current_state, ...
    |                       y_analog, x_analog, obstacle_distances, control_buttons)
    | 
    | braking = BRAKING_TYPE.NONE;
    | next_state = ROVER_STATE.IDLE;
    | 
    | obstacle_left = obstacle_distances(1);
    | obstacle_front = obstacle_distances(2);
    | obstacle_right = obstacle_distances(3);
    | 
    | if y_analog == 0 
    |             
    |     if x_analog > 0 && obstacle_right >= MIN_SIDE_DISTANCE
    |         
    |         next_state = ROVER_STATE.RIGHT;
    | 
    |     elseif x_analog < 0 && obstacle_left >= MIN_SIDE_DISTANCE
    |     
    |         next_state = ROVER_STATE.LEFT;
    | 
    |     else
    |         if bitand(control_buttons, ALT_BACKWARD_MASK) == ALT_BACKWARD_MASK
    |             next_state = ROVER_STATE.ALT_BACKWARD; 
    |         elseif current_state ~= ROVER_STATE.IDLE 
    |             braking = BRAKING_TYPE.HARD;
    |             next_state = ROVER_STATE.IDLE;
    |         else
    |             next_state = ROVER_STATE.IDLE;
    |         end
    | 
    |     end
    | 
    | elseif y_analog < 0
    | 
    |     next_state = ROVER_STATE.BACKWARD;
    | 
    | elseif obstacle_front <= DISTANT_OBSTACLE_DISTANCE 
    |     
    |     if current_state ~= ROVER_STATE.IDLE 
    |         if (obstacle_front <= NEARBY_OBSTACLE_DISTANCE); braking = BRAKING_TYPE.HARD; else; braking = BRAKING_TYPE.SMOOTH;end
    |     end
    |     next_state = ROVER_STATE.IDLE;
    | 
    | elseif x_analog > 0
    |     
    |     if obstacle_right > DISTANT_OBSTACLE_DISTANCE
    | 
    |         next_state = ROVER_STATE.FORWARD_RIGHT;
    | 
    |     else
    |         
    |         braking = BRAKING_TYPE.HARD;
    |         next_state = ROVER_STATE.IDLE;
    | 
    |     end
    | 
    | elseif x_analog < 0
    | 
    |     if obstacle_left > DISTANT_OBSTACLE_DISTANCE
    | 
    |         next_state = ROVER_STATE.FORWARD_LEFT;
    | 
    |     else
    |         
    |         braking = BRAKING_TYPE.HARD;
    |         next_state = ROVER_STATE.IDLE;
    | 
    |     end
    | 
    | elseif y_analog > 0
    | 
    |         next_state = ROVER_STATE.FORWARD;
    | 
    | else 
    |     
    |     braking = BRAKING_TYPE.HARD;
    |     next_state = ROVER_STATE.IDLE;
    | 
    | end
    | 
    | end
  function obstacle = nearby_obstacle_direction(obstacle_distances):
    | function obstacle = nearby_obstacle_direction(obstacle_distances)
    | 
    | obstacle = OBSTACLE_DIR.NOTONE;
    | 
    | obstacle_left = obstacle_distances(1);
    | obstacle_front = obstacle_distances(2);
    | obstacle_right = obstacle_distances(3);
    | 
    | if(obstacle_right <= NEARBY_OBSTACLE_DISTANCE)
    |     if(obstacle_left <= NEARBY_OBSTACLE_DISTANCE)
    |         obstacle = OBSTACLE_DIR.LEFT_RIGHT;
    |     else
    |         obstacle = OBSTACLE_DIR.RIGHT_SIDE;
    |     end
    | elseif(obstacle_left <= NEARBY_OBSTACLE_DISTANCE)
    |     obstacle = OBSTACLE_DIR.LEFT_SIDE;
    | elseif(obstacle_front <= NEARBY_OBSTACLE_DISTANCE)
    |     obstacle = OBSTACLE_DIR.FRONT;
    | end
    | 
    | end
  function joypad_status = check_joypad(control_value, mask):
    | function joypad_status = check_joypad(control_value, mask)
    | 
    | joypad_status = JOYPAD_STATUS.JOYPAD_OK;
    | if bitand(control_value, mask) == 0
    |     joypad_status = JOYPAD_STATUS.JOYPAD_ERR;
    | 
    | end
  function mpu_status = check_mpu(control_value, mask):
    | function mpu_status = check_mpu(control_value, mask)
    | 
    | mpu_status = MPU_STATUS.MPU_OK;
    | if bitand(control_value, mask) == 0
    |     mpu_status = MPU_STATUS.MPU_ERR;
    | 
    | end
